simulink model "W02_1_pose_sub"  (R2024b)
settings: Solver=FixedStepDiscrete  StartTime=0.0  StopTime=inf  FixedStep=Ts  RelTol=1e-3
values from neighbouring files (symbols this model uses):
  Ts = 0.05    [W02_setup.m]
libraries: ros2lib x2
settings Model: Creator=admin  LastModifiedBy=admin

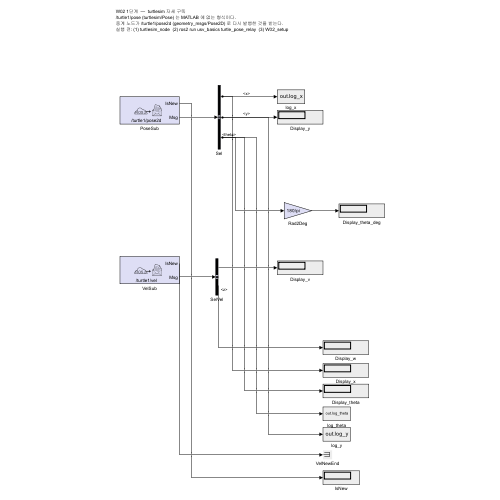
[thumbnail: Simulink's stored preview of the top-level diagram]
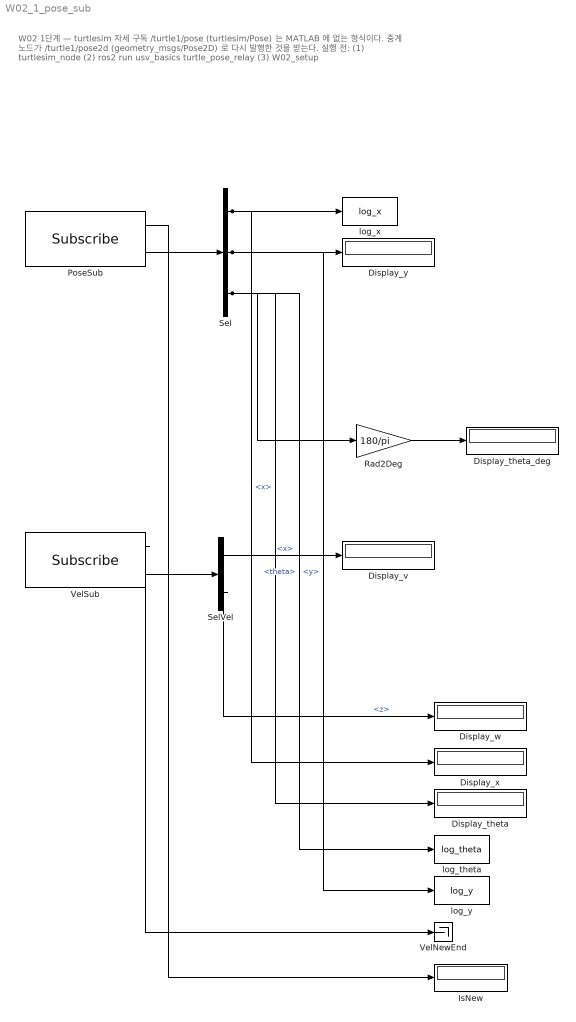
== system W02_1_pose_sub ==
  note: W02 1단계  —  turtlesim 자세 구독
      | /turtle1/pose (turtlesim/Pose) 는 MATLAB 에 없는 형식이다.
      | 중계 노드가 /turtle1/pose2d (geometry_msgs/Pose2D) 로 다시 발행한 것을 받는다.
      | 실행 전: (1) turtlesim_node  (2) ros2 run usv_basics turtle_pose_relay  (3) W02_setup
  Display_theta : Display
  Display_theta_deg : Display
  Display_v : Display
  Display_w : Display
  Display_x : Display
  Display_y : Display
  IsNew : Display
  PoseSub : ros2lib/Subscribe  topicSource=Specify your own  topic=/turtle1/pose2d  messageType=geometry_msgs/Pose2D  sampleTime=Ts  QOSHistory=Keep last  QOSDepth=1  QOSReliability=Reliable  QOSDurability=Volatile  QOSDeadline=Inf  QOSLifespan=Inf  QOSLiveliness=Automatic  QOSLeaseDuration=Inf  QOSAvoidROSNamespaceConventions=off
  Rad2Deg : Gain  Gain=180/pi
  Sel : BusSelector  OutputSignals=x,y,theta
  SelVel : BusSelector  OutputSignals=linear.x,angular.z
  VelNewEnd : Terminator
  VelSub : ros2lib/Subscribe  topicSource=Specify your own  topic=/turtle1/vel  messageType=geometry_msgs/Twist  sampleTime=Ts  QOSHistory=Keep last  QOSDepth=1  QOSReliability=Reliable  QOSDurability=Volatile  QOSDeadline=Inf  QOSLifespan=Inf  QOSLiveliness=Automatic  QOSLeaseDuration=Inf  QOSAvoidROSNamespaceConventions=off
  log_theta : ToWorkspace  VariableName=log_theta  SaveFormat=Timeseries  SampleTime=Ts
  log_x : ToWorkspace  VariableName=log_x  SaveFormat=Timeseries  SampleTime=Ts
  log_y : ToWorkspace  VariableName=log_y  SaveFormat=Timeseries  SampleTime=Ts
  wires:
  SelVel/1 -> Display_v/1  "<x>"
  PoseSub/2 -> Sel/1
  Sel/2 -> Display_y/1, log_y/1  "<y>"
  VelSub/2 -> SelVel/1
  Sel/3 -> Rad2Deg/1, Display_theta/1, log_theta/1  "<theta>"
  Sel/1 -> log_x/1, Display_x/1  "<x>"
  Rad2Deg/1 -> Display_theta_deg/1
  SelVel/2 -> Display_w/1  "<z>"
  VelSub/1 -> VelNewEnd/1
  PoseSub/1 -> IsNew/1
